simulink model "SWC_FDC_type"  (R2021b)
settings: Solver=FixedStepDiscrete  StartTime=0.0  StopTime=10.0  FixedStep=0.001  RelTol=1e-3
values from neighbouring files (symbols this model uses):
  DID_VCUKey = uint16(0x0202)    [vcu_local_hdr.m]
  DID_XWD = uint16(513)    [vcu_local_hdr.m]
  DIDLen_APSFunConfig = uint16(16)    [vcu_local_hdr.m]
  DIDLen_AutoLock = uint16(1)    [vcu_local_hdr.m]
  DIDLen_DKCKey = uint16(8)    [vcu_local_hdr.m]
  DIDLen_DRLDis = uint16(1)    [vcu_local_hdr.m]
  DIDLen_DynoMode = uint16(1)    [vcu_local_hdr.m]
  DIDLen_FMHTimer = uint16(1)    [vcu_local_hdr.m]
  DIDLen_LFLowPresThre = uint16(1)    [vcu_local_hdr.m]
  DIDLen_LFSensorID = uint16(4)    [vcu_local_hdr.m]
  DIDLen_LRLowPresThre = uint16(1)    [vcu_local_hdr.m]
  DIDLen_LRSensorID = uint16(4)    [vcu_local_hdr.m]
  DIDLen_RFLowPresThre = uint16(1)    [vcu_local_hdr.m]
  DIDLen_RFSensorID = uint16(4)    [vcu_local_hdr.m]
  DIDLen_RRLowPresThre = uint16(1)    [vcu_local_hdr.m]
  DIDLen_RRSensorID = uint16(4)    [vcu_local_hdr.m]
  DIDLen_SensorMode = uint16(1)    [vcu_local_hdr.m]
  DIDLen_TireSize = uint16(16)    [vcu_local_hdr.m]
  DIDLen_TPMSLearnSta = uint16(1)    [vcu_local_hdr.m]
  DIDLen_TurnLampFLThreCurr = uint16(1)    [vcu_local_hdr.m]
  DIDLen_TurnLampFRThreCurr = uint16(1)    [vcu_local_hdr.m]
  DIDLen_TurnLampRLThreCurr = uint16(1)    [vcu_local_hdr.m]
  DIDLen_TurnLampRRThreCurr = uint16(1)    [vcu_local_hdr.m]
  DIDLen_USSConfig = uint16(16)    [vcu_local_hdr.m]
  DIDLen_WhlPres = uint16(4)    [vcu_local_hdr.m]
  DIDLen_WhlSensorBattSta = uint16(1)    [vcu_local_hdr.m]
  DIDLen_WhlTmp = uint16(4)    [vcu_local_hdr.m]
  DIDLen_XWDMode = uint16(1)    [vcu_local_hdr.m]
  DIDNum_APSFunConfig = uint16(0x0903)    [vcu_local_hdr.m]
  DIDNum_AutoLock = uint16(0x0306)    [vcu_local_hdr.m]
  DIDNum_DKCKey = uint16(0x0202)    [vcu_local_hdr.m]
  DIDNum_DRLDis = uint16(0x0307)    [vcu_local_hdr.m]
  DIDNum_DynoMode = uint16(0x0203)    [vcu_local_hdr.m]
  DIDNum_FMHTimer = uint16(0x0305)    [vcu_local_hdr.m]
  DIDNum_LFLowPresThre = uint16(0x0B08)    [vcu_local_hdr.m]
  DIDNum_LFSensorID = uint16(0x0B01)    [vcu_local_hdr.m]
  DIDNum_LRLowPresThre = uint16(0x0B0A)    [vcu_local_hdr.m]
  DIDNum_LRSensorID = uint16(0x0B03)    [vcu_local_hdr.m]
  DIDNum_RFLowPresThre = uint16(0x0B09)    [vcu_local_hdr.m]
  DIDNum_RFSensorID = uint16(0x0B02)    [vcu_local_hdr.m]
  DIDNum_RRLowPresThre = uint16(0x0B0B)    [vcu_local_hdr.m]
  DIDNum_RRSensorID = uint16(0x0B04)    [vcu_local_hdr.m]
  DIDNum_SensorMode = uint16(0x0B0C)    [vcu_local_hdr.m]
  DIDNum_TireSize = uint16(0x0902)    [vcu_local_hdr.m]
  DIDNum_TPMSLearnSta = uint16(0x0B0D)    [vcu_local_hdr.m]
  DIDNum_TurnLampFLThreCurr = uint16(0x0303)    [vcu_local_hdr.m]
  DIDNum_TurnLampFRThreCurr = uint16(0x0301)    [vcu_local_hdr.m]
  DIDNum_TurnLampRLThreCurr = uint16(0x0304)    [vcu_local_hdr.m]
  DIDNum_TurnLampRRThreCurr = uint16(0x0302)    [vcu_local_hdr.m]
  DIDNum_USSConfig = uint16(0x0901)    [vcu_local_hdr.m]
  DIDNum_WhlPres = uint16(0x0B05)    [vcu_local_hdr.m]
  DIDNum_WhlSensorBattSta = uint16(0x0B07)    [vcu_local_hdr.m]
  DIDNum_WhlTmp = uint16(0x0B06)    [vcu_local_hdr.m]
  DIDNum_XWDMode = uint16(0x0201)    [vcu_local_hdr.m]
  DIDVCUKeyLength = uint16(8)    [vcu_local_hdr.m]
  ENUM_DRIVETRAIN_AWD = uint8(  2  )    [vcu_local_hdr.m]
  ENUM_DRIVETRAIN_FWD = uint8(  1  )    [vcu_local_hdr.m]
  ENUM_DRIVETRAIN_RWD = uint8(  0  )    [vcu_local_hdr.m]
  ENUM_TPMSLearnStatus_LEARNED = uint8(  1  )    [vcu_local_hdr.m]
  ENUM_TPMSLearnStatus_LEARNFAIL = uint8(  2  )    [vcu_local_hdr.m]
  ENUM_TPMSLearnStatus_NOTLEARN = uint8(  0  )    [vcu_local_hdr.m]
  ENUM_TPMSSTA_FAT = uint8(  8  )    [vcu_local_hdr.m]
  ENUM_TPMSSTA_LOWBATTERY = uint8(  2  )    [vcu_local_hdr.m]
  FALSE = boolean( 0 )    [vcu_local_hdr.m]
  ONE_INT = uint8(1)    [vcu_local_hdr.m]
  P_boolean = 0.0    [APPTypes.sldd]
  TRUE = boolean( 1 )    [vcu_local_hdr.m]
  ZERO_FLOAT = single(0)    [vcu_local_hdr.m]
  ZERO_INT = uint8(0)    [vcu_local_hdr.m]
undefined symbols (not defined in the file or in its folder): f32_ApsOutVehSpdSig, KHAL_DKCDecryptEnable_flg_ovrdflg, KHAL_DKCDecryptEnable_flg_ovrdval, KHAL_RandomNumberY1_enum, KHAL_RandomNumberY2_enum, KHAL_RandomNumberY_ovrdflg, KHAL_TPMSRESBUTT_flg_ovrdflg, KHAL_TPMSRESBUTT_flg_ovrdval, R_DIDWriteCDD_CSOP_DIDSet_APSFunConfig, R_DIDWriteCDD_CSOP_DIDSet_AutoLock, R_DIDWriteCDD_CSOP_DIDSet_DKCKey, R_DIDWriteCDD_CSOP_DIDSet_DRLDis, R_DIDWriteCDD_CSOP_DIDSet_DynoMode, R_DIDWriteCDD_CSOP_DIDSet_FMHTimer, R_DIDWriteCDD_CSOP_DIDSet_LFLowPresThre, R_DIDWriteCDD_CSOP_DIDSet_LFSensorID, R_DIDWriteCDD_CSOP_DIDSet_LRLowPresThre, R_DIDWriteCDD_CSOP_DIDSet_LRSensorID, R_DIDWriteCDD_CSOP_DIDSet_RFLowPresThre, R_DIDWriteCDD_CSOP_DIDSet_RFSensorID, R_DIDWriteCDD_CSOP_DIDSet_RRLowPresThre, R_DIDWriteCDD_CSOP_DIDSet_RRSensorID, R_DIDWriteCDD_CSOP_DIDSet_SensorMode, R_DIDWriteCDD_CSOP_DIDSet_TireSize, R_DIDWriteCDD_CSOP_DIDSet_TPMSLearnSta, R_DIDWriteCDD_CSOP_DIDSet_TurnLampFLThreCurr, R_DIDWriteCDD_CSOP_DIDSet_TurnLampFRThreCurr, R_DIDWriteCDD_CSOP_DIDSet_TurnLampRLThreCurr, R_DIDWriteCDD_CSOP_DIDSet_TurnLampRRThreCurr, R_DIDWriteCDD_CSOP_DIDSet_USSConfig, R_DIDWriteCDD_CSOP_DIDSet_WhlPres, R_DIDWriteCDD_CSOP_DIDSet_WhlSensorBattSta, R_DIDWriteCDD_CSOP_DIDSet_WhlTmp, R_DIDWriteCDD_CSOP_DIDSet_XWDMode, R_E2E_CAN3_VCU1_CSOP_Write_CAN3_VCU1, R_E2E_CAN3_VCU1_toNIDEC_CSOP_Write_CAN3_VCU1_toNIDEC, R_E2E_CAN4_VCU1_CSOP_Write_CAN4_VCU1, R_FDCCDD_Inner_CSOP_FDC_AppCallSleep, R_HALINCDD_CSOP_PAS_Handler, R_HALINCDD_CSOP_UDS_Main, R_HALOUT_APS_CSOP_ApsOutput, R_HALOUTCDD_CSOP_AppNmStateReq, R_HALOUTCDD_CSOP_SetAcoreRebootCmdACK, R_HALOUTCDD_CSOP_SetSysPwrStat, R_HALOUTCDD_CSOP_SleepRequest, R_IOExpOUT_CDD_CSOP_IOExpSetVal, R_J1939_CAN1_CFGEM1_BAM_CSOP_Write_CAN1_CFGEM1_BAM, R_J1939_CAN1_CFGEM1_DT_CSOP_Write_CAN1_CFGEM1_DT, R_NVMReadCDD_Inner_NVM_ReadOperation, R_NVMWriteCDD_Inner_NVM_WriteOperation, R_UDSCDD_CSOP_DdmRestartOperationCycle, R_WDGCDD_CSOP_Call_Watchdog, R_WDGCDD_CSOP_Call_WDG_AppEnd, R_WDGCDD_CSOP_Call_WDG_AppStart, u16_DIDLen_APSFunConfig, u16_DIDLen_AutoLock, u16_DIDLen_DKCKey, u16_DIDLen_DRLDis, u16_DIDLen_DynoMode, u16_DIDLen_FMHTimer ... (+83)
libraries: simulink x215, FVT_lib x143, hcu_lib x19, hdlsllib x9, app x1, halin x1, halout x1, inp x1, outp x1
(part 3 of 13)

== system SWC_FDC_type/run_SWC_FDC_Tx_10ms_sys ==
  IRV_ms10_CAN1_SG_EMRC1_read : Inport
  IRV_ms10_CAN1_SG_VCU_PDU_Demand_1_read : Inport  Port=2
  IRV_ms10_CAN2_SG_GW2_C10_0_read : Inport  Port=3
  IRV_ms10_CAN3_SG_FD3_VCU0_read : Inport  Port=4
  IRV_ms10_CAN3_SG_FD3_VCU2_read : Inport  Port=5
  IRV_ms10_CAN3_SG_FD3_VCU2_toNIDEC_read : Inport  Port=6
  IRV_ms10_CAN3_SG_FD3_VCU5_read : Inport  Port=7
  IRV_f32_ApsOutVehSpdSig_read : Inport  Port=8
  IRV_u8_ApsOutGearPosnSig_read : Inport  Port=9
  IRV_u8_ApsOutSendChrgPlugSta_read : Inport  Port=10
  IRV_u8_ApsOutSetFrSensorOnCmd_read : Inport  Port=11
  IRV_u8_ApsOutSetFrSensorSwTOCmd_read : Inport  Port=12
  IRV_u8_ApsOutSetVehSpdTOCmd_read : Inport  Port=13
  function : TriggerPort  TriggerType=function-call  VariantControl=(inherit)  SampleTimeType=periodic  SampleTime=-1
  R_HALINCDD_CSOP_TPMS_GetRawData : FunctionCaller  FunctionPrototype=[u8_TPMSDataInSta,u8Array9_TPMSData] = R_HALINCDD_CSOP_TPMS_GetRawData()  OutputArgumentSpecifications=P_boolean, uint8([1;1;1;1;1;1;1;1;1])
  R_HALIN_APS_CSOP_ApsGetDist : FunctionCaller  FunctionPrototype=[u8Array8_PasInDist,u16Array4_ApsInDist] = R_HALIN_APS_CSOP_ApsGetDist()  OutputArgumentSpecifications=uint8([1;1;1;1;1;1;1;1]), uint16([1;1;1;1])
  R_HALIN_APS_CSOP_ApsGetDistLevel : FunctionCaller  FunctionPrototype=u8Array8_ApsInLevel = R_HALIN_APS_CSOP_ApsGetDistLevel()  OutputArgumentSpecifications=uint8([1;1;1;1;1;1;1;1])
  R_HALIN_APS_CSOP_ApsGetOtherStatus : FunctionCaller  FunctionPrototype=[u8_ApsInPASChime,u8_ApsInSensorLayout,u8_ApsInSysFailSta,u8_ApsInSysMode] = R_HALIN_APS_CSOP_ApsGetOtherStatus()  OutputArgumentSpecifications=uint8(1), uint8(1), uint8(1), uint8(1)
  R_HALIN_APS_CSOP_ApsGetUssSta : FunctionCaller  FunctionPrototype=u8Array12_ApsInUssSta = R_HALIN_APS_CSOP_ApsGetUssSta()  OutputArgumentSpecifications=uint8([1;1;1;1;1;1;1;1;1;1;1;1])
  R_HALOUT_APS_CSOP_ApsOutput : FunctionCaller  FunctionPrototype=R_HALOUT_APS_CSOP_ApsOutput(f32_ApsOutVehSpdSig,u8_ApsOutGearPosnSig,u8_ApsOutSetFrSensorOnCmd,u8_ApsOutSetVehSpdTOCmd,u8_ApsOutSetFrSensorSwTOCmd,u8_ApsOutSendChrgPlugSta)  InputArgumentSpecifications=single(1), uint8(1), uint8(1), uint8(1), uint8(1), uint8(1)
  P_CAN1_EMRC1_CAN1_SG_EMRC1_write : Outport
  P_CAN1_VCU_PDU_Demand_1_CAN1_SG_VCU_PDU_Demand_1_write : Outport  Port=2
  P_CAN2_GW2_C10_0_CAN2_SG_GW2_C10_0_write : Outport  Port=3
  P_CAN3_FD3_VCU0_CAN3_SG_FD3_VCU0_write : Outport  Port=4
  P_CAN3_FD3_VCU2_CAN3_SG_FD3_VCU2_write : Outport  Port=5
  P_CAN3_FD3_VCU2_toNIDEC_CAN3_SG_FD3_VCU2_toNIDEC_write : Outport  Port=6
  P_CAN3_FD3_VCU5_CAN3_SG_FD3_VCU5_write : Outport  Port=7
  IRV_u16Array4_ApsInDist_write : Outport  Port=8  OutDataTypeStr=uint16  PortDimensions=4
  IRV_u8Array12_ApsInUssSta_write : Outport  Port=9  OutDataTypeStr=uint8  PortDimensions=12
  IRV_u8Array8_ApsInLevel_write : Outport  Port=10  OutDataTypeStr=uint8  PortDimensions=8
  IRV_u8Array8_PasInDist_write : Outport  Port=11  OutDataTypeStr=uint8  PortDimensions=8
  IRV_u8Array9_TPMSData_write : Outport  Port=12  OutDataTypeStr=uint8  PortDimensions=9
  IRV_u8_ApsInPASChime_write : Outport  Port=13  OutDataTypeStr=uint8  PortDimensions=1
  IRV_u8_ApsInSensorLayout_write : Outport  Port=14  OutDataTypeStr=uint8  PortDimensions=1
  IRV_u8_ApsInSysFailSta_write : Outport  Port=15  OutDataTypeStr=uint8  PortDimensions=1
  IRV_u8_ApsInSysMode_write : Outport  Port=16  OutDataTypeStr=uint8  PortDimensions=1
  IRV_u8_TPMSDataInSta_write : Outport  Port=17  OutDataTypeStr=uint8  PortDimensions=1
  wires:
  R_HALIN_APS_CSOP_ApsGetDist/1 -> IRV_u8Array8_PasInDist_write/1
  R_HALIN_APS_CSOP_ApsGetDist/2 -> IRV_u16Array4_ApsInDist_write/1
  R_HALIN_APS_CSOP_ApsGetDistLevel/1 -> IRV_u8Array8_ApsInLevel_write/1
  R_HALIN_APS_CSOP_ApsGetUssSta/1 -> IRV_u8Array12_ApsInUssSta_write/1
  IRV_f32_ApsOutVehSpdSig_read/1 -> R_HALOUT_APS_CSOP_ApsOutput/1
  IRV_u8_ApsOutGearPosnSig_read/1 -> R_HALOUT_APS_CSOP_ApsOutput/2
  IRV_u8_ApsOutSetFrSensorOnCmd_read/1 -> R_HALOUT_APS_CSOP_ApsOutput/3
  IRV_u8_ApsOutSetVehSpdTOCmd_read/1 -> R_HALOUT_APS_CSOP_ApsOutput/4
  IRV_u8_ApsOutSetFrSensorSwTOCmd_read/1 -> R_HALOUT_APS_CSOP_ApsOutput/5
  IRV_u8_ApsOutSendChrgPlugSta_read/1 -> R_HALOUT_APS_CSOP_ApsOutput/6
  R_HALIN_APS_CSOP_ApsGetOtherStatus/1 -> IRV_u8_ApsInPASChime_write/1
  R_HALIN_APS_CSOP_ApsGetOtherStatus/2 -> IRV_u8_ApsInSensorLayout_write/1
  R_HALIN_APS_CSOP_ApsGetOtherStatus/3 -> IRV_u8_ApsInSysFailSta_write/1
  R_HALIN_APS_CSOP_ApsGetOtherStatus/4 -> IRV_u8_ApsInSysMode_write/1
  R_HALINCDD_CSOP_TPMS_GetRawData/1 -> IRV_u8_TPMSDataInSta_write/1
  R_HALINCDD_CSOP_TPMS_GetRawData/2 -> IRV_u8Array9_TPMSData_write/1
  IRV_ms10_CAN1_SG_EMRC1_read/1 -> P_CAN1_EMRC1_CAN1_SG_EMRC1_write/1
  IRV_ms10_CAN1_SG_VCU_PDU_Demand_1_read/1 -> P_CAN1_VCU_PDU_Demand_1_CAN1_SG_VCU_PDU_Demand_1_write/1
  IRV_ms10_CAN2_SG_GW2_C10_0_read/1 -> P_CAN2_GW2_C10_0_CAN2_SG_GW2_C10_0_write/1
  IRV_ms10_CAN3_SG_FD3_VCU0_read/1 -> P_CAN3_FD3_VCU0_CAN3_SG_FD3_VCU0_write/1
  IRV_ms10_CAN3_SG_FD3_VCU2_toNIDEC_read/1 -> P_CAN3_FD3_VCU2_toNIDEC_CAN3_SG_FD3_VCU2_toNIDEC_write/1
  IRV_ms10_CAN3_SG_FD3_VCU5_read/1 -> P_CAN3_FD3_VCU5_CAN3_SG_FD3_VCU5_write/1
  IRV_ms10_CAN3_SG_FD3_VCU2_read/1 -> P_CAN3_FD3_VCU2_CAN3_SG_FD3_VCU2_write/1

== system SWC_FDC_type/run_SWC_FDC_Tx_20ms_sys ==
  IRV_ms20_CAN2_SG_FD2_C20_0_read : Inport
  function : TriggerPort  TriggerType=function-call  VariantControl=(inherit)  SampleTimeType=periodic  SampleTime=-1
  P_CAN2_FD2_C20_0_CAN2_SG_FD2_C20_0_write : Outport
  wires:
  IRV_ms20_CAN2_SG_FD2_C20_0_read/1 -> P_CAN2_FD2_C20_0_CAN2_SG_FD2_C20_0_write/1

== system SWC_FDC_type/run_SWC_FDC_Tx_250ms_sys ==
  IRV_ms250_CAN1_SG_EEC3_read : Inport
  function : TriggerPort  TriggerType=function-call  VariantControl=(inherit)  SampleTimeType=periodic  SampleTime=-1
  P_CAN1_EEC3_CAN1_SG_EEC3_write : Outport
  wires:
  IRV_ms250_CAN1_SG_EEC3_read/1 -> P_CAN1_EEC3_CAN1_SG_EEC3_write/1

== system SWC_FDC_type/run_SWC_FDC_Tx_5000ms_sys ==
  IRV_ms5000_CAN2_SG_FD2_Version_read : Inport
  function : TriggerPort  TriggerType=function-call  VariantControl=(inherit)  SampleTimeType=periodic  SampleTime=-1
  P_CAN2_FD2_Version_CAN2_SG_FD2_Version_write : Outport
  wires:
  IRV_ms5000_CAN2_SG_FD2_Version_read/1 -> P_CAN2_FD2_Version_CAN2_SG_FD2_Version_write/1

== system SWC_FDC_type/run_SWC_FDC_Tx_50ms_sys ==
  IRV_ms50_CAN1_SG_EEC2_read : Inport
  IRV_ms50_CAN1_SG_ETC2_read : Inport  Port=2
  function : TriggerPort  TriggerType=function-call  VariantControl=(inherit)  SampleTimeType=periodic  SampleTime=-1
  P_CAN1_EEC2_CAN1_SG_EEC2_write : Outport
  P_CAN1_ETC2_CAN1_SG_ETC2_write : Outport  Port=2
  wires:
  IRV_ms50_CAN1_SG_EEC2_read/1 -> P_CAN1_EEC2_CAN1_SG_EEC2_write/1
  IRV_ms50_CAN1_SG_ETC2_read/1 -> P_CAN1_ETC2_CAN1_SG_ETC2_write/1

== system SWC_FDC_type/run_SWC_FDC_Tx_80ms_sys ==
  IRV_ms80_CAN1_SG_ETC1_read : Inport
  function : TriggerPort  TriggerType=function-call  VariantControl=(inherit)  SampleTimeType=periodic  SampleTime=-1
  P_CAN1_ETC1_CAN1_SG_ETC1_write : Outport
  wires:
  IRV_ms80_CAN1_SG_ETC1_read/1 -> P_CAN1_ETC1_CAN1_SG_ETC1_write/1

== system SWC_FDC_type/run_SWC_FDC_UDS_10ms_sys ==
  function : TriggerPort  TriggerType=function-call  VariantControl=(inherit)  SampleTimeType=periodic  SampleTime=-1
  R_HALINCDD_CSOP_UDS_Main : FunctionCaller  FunctionPrototype=R_HALINCDD_CSOP_UDS_Main()

== system SWC_FDC_type/P_WDGCDD/run_SWC_FDC_AppCallWDG_End_sys ==
  function : TriggerPort  TriggerType=function-call  IsSimulinkFunction=on  FunctionName=run_SWC_FDC_AppCallWDG_End  VariantControl=(inherit)

== system SWC_FDC_type/P_WDGCDD/run_SWC_FDC_AppCallWDG_StartUp_sys ==
  function : TriggerPort  TriggerType=function-call  IsSimulinkFunction=on  FunctionName=run_SWC_FDC_AppCallWDG_StartUp  VariantControl=(inherit)

== system SWC_FDC_type/P_WDGCDD/run_SWC_FDC_AppCallWDG_sys ==
  function : TriggerPort  TriggerType=function-call  IsSimulinkFunction=on  FunctionName=run_SWC_FDC_AppCallWDG  VariantControl=(inherit)

== system SWC_FDC_type/run_SWC_FDC_RxTx_5ms_sys/HALOUT_AFTER ==
  E2E_CAN3_VCU1_Trigger : Inport
  E2E_CAN3_VCU1_Trigger_toNIDEC : Inport  Port=2
  E2E_CAN4_VCU1_Trigger : Inport  Port=3
  function : TriggerPort  TriggerType=function-call  VariantControl=(inherit)  PortDimensions=1
  R_E2E_CAN3_VCU1_CSOP_Write_CAN3_VCU1 : Subsystem
  R_E2E_CAN3_VCU1_toNIDEC_CSOP_Write_CAN3_VCU1_toNIDEC : Subsystem
  R_E2E_CAN4_VCU1_CSOP_Write_CAN4_VCU1 : Subsystem
  wires:
  E2E_CAN3_VCU1_Trigger/1 -> R_E2E_CAN3_VCU1_CSOP_Write_CAN3_VCU1/Enable
  E2E_CAN3_VCU1_Trigger_toNIDEC/1 -> R_E2E_CAN3_VCU1_toNIDEC_CSOP_Write_CAN3_VCU1_toNIDEC/Enable
  E2E_CAN4_VCU1_Trigger/1 -> R_E2E_CAN4_VCU1_CSOP_Write_CAN4_VCU1/Enable

== system SWC_FDC_type/run_SWC_FDC_RxTx_5ms_sys/Halin_CDD ==
  PASDistanceData : Inport
  APSDistanceData : Inport  Port=2
  APSLevelData : Inport  Port=3
  APSFaultStaData : Inport  Port=4
  ChimeIn : Inport  Port=5
  SNSRLayoutIn : Inport  Port=6
  StaFSyaIn : Inport  Port=7
  ModOperationIn : Inport  Port=8
  VHAL_AccelPedal1Vol_Raw : Inport  Port=9
  VHAL_AccelPedal2Vol_Raw : Inport  Port=10
  VHAL_BrakeSWGPIO_flg : Inport  Port=11
  VHAL_HoodSW_flg : Inport  Port=12
  VHAL_TailgateSW_flg : Inport  Port=13
  VHAL_DrDoorSW_flg : Inport  Port=14
  VHAL_PsDoorSW_flg : Inport  Port=15
  VHAL_RRDoorSW_flg : Inport  Port=16
  VHAL_RLDoorSW_flg : Inport  Port=17
  VHAL_CentralDoorLockSW_flg : Inport  Port=18
  VHAL_HazardSW_flg : Inport  Port=19
  VHAL_BrakeLampSW_flg : Inport  Port=20
  VHAL_TrunkHanSW_flg : Inport  Port=21
  VHAL_SeatSW_flg : Inport  Port=22
  VHAL_CrashSignalGPIO_flg : Inport  Port=23
  u8_HWID_4byte : Inport  Port=24
  GetSWID_status : Inport  Port=25
  GetSWID_data : Inport  Port=26
  VHAL_AnyNMID_flg : Inport  Port=27
  VHAL_CurrentNmState_enum : Inport  Port=28
  VHAL_PwrReq_OTA_enum : Inport  Port=29
  VHAL_AllowMovThd_OTA_enum : Inport  Port=30
  VHAL_EvccAplusPwrUpReq_flg : Inport  Port=31
  VHAL_AcoreReadyToSlp_flg : Inport  Port=32
  VHAL_DidXWDSta_flg : Inport  Port=33
  VHAL_DidXWDData_enum : Inport  Port=34
  HAL_NvmReadData_raw : Inport  Port=35
  VHAL_DIDVCUKeyReadSta_flg : Inport  Port=36
  VHAL_GetDIDVCUKey_enum : Inport  Port=37
  TPMS_DataIn_flg : Inport  Port=38
  TPMS_RawData : Inport  Port=39
  BHAL_CAN2_outputs : Inport  Port=40
  BHAL_CAN4_outputs : Inport  Port=41
  VHAL_ClearDTCcmd_flg : Inport  Port=42
  VHAL_IMUOffsetVal_raw : Inport  Port=43
  VHAL_IMUSixAxisVal_raw : Inport  Port=44
  VHAL_IMUOffsetValSta_flg : Inport  Port=45
  VHAL_IMUSixAxisValSta_flg : Inport  Port=46
  VHAL_NvmProtectSta_flg : Inport  Port=47
  VHAL_AuxBattVolmV_100mV : Inport  Port=48
  VHAL_Pedal1Ref5V_raw : Inport  Port=49
  VHAL_Pedal2Ref5V_raw : Inport  Port=50
  VHAL_NetworkReqCalled_flg : Inport  Port=51
  VHAL_PmicBootReason_enum : Inport  Port=52
  VHAL_WisrBootReason_raw32 : Inport  Port=53
  BHAL_DIDGetData_raw : Inport  Port=54
  VHAL_AcoreRebootCmd_raw : Inport  Port=55
  VHAL_CAN1BusOff_raw : Inport  Port=56
  VHAL_CAN2BusOff_raw : Inport  Port=57
  VHAL_CAN3BusOff_raw : Inport  Port=58
  VHAL_CAN4BusOff_raw : Inport  Port=59
  VHAL_CAN5BusOff_raw : Inport  Port=60
  u8_GetAPS_Progress_PCT : Inport  Port=61
  u8_GetAPS_RQ_Display : Inport  Port=62
  u8_GetAPS_SW_Ver : Inport  Port=63
  u8_GetAPS_HW_Ver : Inport  Port=64
  u8_GetAPS_ExitCondition : Inport  Port=65
  f32_GetAPS_Angle_Target : Inport  Port=66
  u8_GetAPS_Sta_System : Inport  Port=67
  u8_GetAPS_V_Rq_EPAS_Ctrl : Inport  Port=68
  u8_GetAPS_Rq_EPAS_Ctrl : Inport  Port=69
  u8_GetAPS_Req : Inport  Port=70
  f32_GetAPS_DecReq : Inport  Port=71
  u8_GetAPS_DecReq_A : Inport  Port=72
  f32_GetAPS_SpeedCmd : Inport  Port=73
  u8_GetAPS_ShftPosnReq : Inport  Port=74
  u8_GetAPS_VMC_Req_A : Inport  Port=75
  u8_GetCAAS_Sta : Inport  Port=76
  u8_GetCAAS_VMC_Req_A : Inport  Port=77
  trig_HalinCDD : TriggerPort  TriggerType=function-call  VariantControl=(inherit)
  Halin_APM : Subsystem
  Halin_DKC_A : Subsystem
  Halin_GPIO : Subsystem
  Halin_IMU : Subsystem
  Halin_SYS : Subsystem
  Halin_TPMS : Subsystem
  Subsystem : Subsystem
  TPM_Scheduler : Stateflow chart  TreatAsAtomicUnit=on
  BHAL_APM_outputs : Outport
  BHAL_GPIO_outputs : Outport  Port=2
  BHAL_SYS_outputs : Outport  Port=3
  BHAL_TPMS_outputs : Outport  Port=4
  BHAL_SYSTPMS_outputs : Outport  Port=5
  BHAL_DDM_outputs : Outport  Port=6
  BHAL_IMU_outputs : Outport  Port=7
  Enable_decrypt : Outport  Port=8
  AESKey : Outport  Port=9
  DKCRawData : Outport  Port=10
  wires:
  Halin_DKC_A/1(Enable_Decrypt) -> Enable_decrypt/1
  VHAL_RLDoorSW_flg/1 -> Halin_GPIO/9(VHAL_RLDoorSW_flg)
  Halin_SYS/1(BHAL_SYS_outputs) -> [BHAL_SYS_outputs], BHAL_SYS_outputs/1
  Halin_DKC_A/3(DKCRawData) -> DKCRawData/1
  GetSWID_data/1 -> Halin_SYS/2(GetSWID_data)
  VHAL_GetDIDVCUKey_enum/1 -> Halin_SYS/13(VHAL_GetDIDVCUKey_enum)
  VHAL_TailgateSW_flg/1 -> Halin_GPIO/5(VHAL_TailgateSW_flg)
  Halin_DKC_A/2(AESKey) -> AESKey/1
  VHAL_AccelPedal2Vol_Raw/1 -> Halin_GPIO/2(VHAL_AccelPedal2Vol_Raw)
  TPM_Scheduler/1(trig_TPM_10ms1()) -> Halin_TPMS/Trigger
  VHAL_TrunkHanSW_flg/1 -> Halin_GPIO/13(VHAL_TrunkHanSW_flg)
  VHAL_DidXWDSta_flg/1 -> Halin_SYS/9(VHAL_DidXWDSta_flg)
  VHAL_CurrentNmState_enum/1 -> Halin_SYS/4(VHAL_CurrentNmState_enum)
  VHAL_AccelPedal1Vol_Raw/1 -> Halin_GPIO/1(VHAL_AccelPedal1Vol_Raw)
  u8_HWID_4byte/1 -> Halin_GPIO/16(u8_HWID_4byte)
  BHAL_CAN2_outputs/1 -> Halin_TPMS/3(BHAL_CAN2_outputs)
  VHAL_AcoreReadyToSlp_flg/1 -> Halin_SYS/8(VHAL_AcoreReadyToSlp_flg)
  HAL_NvmReadData_raw/1 -> Halin_SYS/11(HAL_NvmReadData_raw)
  VHAL_AllowMovThd_OTA_enum/1 -> Halin_SYS/6(VHAL_AllowMovThd_OTA_enum)
  VHAL_BrakeLampSW_flg/1 -> Halin_GPIO/12(VHAL_BrakeLampSW_flg)
  VHAL_RRDoorSW_flg/1 -> Halin_GPIO/8(VHAL_RRDoorSW_flg)
  VHAL_BrakeSWGPIO_flg/1 -> Halin_GPIO/3(VHAL_BrakeSWGPIO_flg)
  GetSWID_status/1 -> Halin_SYS/1(GetSWID_status)
  VHAL_DrDoorSW_flg/1 -> Halin_GPIO/6(VHAL_DrDoorSW_flg)
  VHAL_PwrReq_OTA_enum/1 -> Halin_SYS/5(VHAL_PwrReq_OTA_enum)
  VHAL_HoodSW_flg/1 -> Halin_GPIO/4(VHAL_HoodSW_flg)
  Halin_GPIO/1(BHAL_GPIO_outputs) -> BHAL_GPIO_outputs/1
  BHAL_CAN4_outputs/1 -> Halin_DKC_A/1(BHAL_CAN4_outputs)
  VHAL_CentralDoorLockSW_flg/1 -> Halin_GPIO/10(VHAL_CentralDoorLockSW_flg)
  TPMS_RawData/1 -> Halin_TPMS/2(TPMS_RawData)
  VHAL_CrashSignalGPIO_flg/1 -> Halin_GPIO/15(VHAL_CrashSignalGPIO_flg)
  Halin_TPMS/1(BHAL_TPMS_outputs) -> BHAL_TPMS_outputs/1
  VHAL_DidXWDData_enum/1 -> Halin_SYS/10(VHAL_DidXWDData_enum)
  VHAL_EvccAplusPwrUpReq_flg/1 -> Halin_SYS/7(VHAL_EvccAplusPwrUpReq_flg)
  VHAL_SeatSW_flg/1 -> Halin_GPIO/14(VHAL_SeatSW_flg)
  VHAL_DIDVCUKeyReadSta_flg/1 -> Halin_SYS/12(VHAL_DIDVCUKeyReadSta_flg)
  VHAL_PsDoorSW_flg/1 -> Halin_GPIO/7(VHAL_PsDoorSW_flg)
  [BHAL_SYS_outputs] -> Halin_DKC_A/2(BHAL_SYS_outputs)
  TPMS_DataIn_flg/1 -> Halin_TPMS/1(TPMS_DataIn_flg)
  VHAL_AnyNMID_flg/1 -> Halin_SYS/3(VHAL_AnyNMID_flg)
  VHAL_HazardSW_flg/1 -> Halin_GPIO/11(VHAL_HazardSW_flg)
  Halin_SYS/2(BHAL_SYSTPMS_outputs) -> [BHAL_SYSTPMS_outputs], BHAL_SYSTPMS_outputs/1
  [BHAL_SYSTPMS_outputs] -> Halin_TPMS/4(BHAL_SYSTPMS_outputs)
  VHAL_ClearDTCcmd_flg/1 -> Subsystem/1(VHAL_ClearDTCcmd_flg)
  Subsystem/1(BHAL_DDM_outputs) -> BHAL_DDM_outputs/1
  Halin_IMU/1(BHAL_IMU_outputs) -> BHAL_IMU_outputs/1
  VHAL_IMUOffsetVal_raw/1 -> Halin_IMU/1(VHAL_IMUOffsetVal_raw)
  VHAL_IMUOffsetValSta_flg/1 -> Halin_IMU/3(VHAL_IMUOffsetValSta_flg)
  VHAL_IMUSixAxisVal_raw/1 -> Halin_IMU/2(VHAL_IMUSixAxisVal_raw)
  VHAL_IMUSixAxisValSta_flg/1 -> Halin_IMU/4(VHAL_IMUSixAxisValSta_flg)
  VHAL_NvmProtectSta_flg/1 -> Halin_SYS/14(VHAL_NvmProtectSta_flg)
  VHAL_AuxBattVolmV_100mV/1 -> Halin_SYS/15(VHAL_AuxBattVolmV_100mV)
  VHAL_Pedal1Ref5V_raw/1 -> Halin_SYS/16(VHAL_Pedal1Ref5V_raw)
  VHAL_Pedal2Ref5V_raw/1 -> Halin_SYS/17(VHAL_Pedal2Ref5V_raw)
  VHAL_NetworkReqCalled_flg/1 -> Halin_SYS/18(VHAL_NetworkReqCalled_flg)
  VHAL_PmicBootReason_enum/1 -> Halin_SYS/19(VHAL_PmicBootReason_enum)
  VHAL_WisrBootReason_raw32/1 -> Halin_SYS/20(VHAL_WisrBootReason_raw32)
  BHAL_DIDGetData_raw/1 -> Halin_SYS/21(BHAL_DIDGetData_raw)
  VHAL_AcoreRebootCmd_raw/1 -> Halin_SYS/22(VHAL_AcoreRebootCmd_raw)
  VHAL_CAN1BusOff_raw/1 -> Halin_SYS/23(VHAL_CAN1BusOff_raw)
  VHAL_CAN2BusOff_raw/1 -> Halin_SYS/24(VHAL_CAN2BusOff_raw)
  VHAL_CAN3BusOff_raw/1 -> Halin_SYS/25(VHAL_CAN3BusOff_raw)
  VHAL_CAN4BusOff_raw/1 -> Halin_SYS/26(VHAL_CAN4BusOff_raw)
  VHAL_CAN5BusOff_raw/1 -> Halin_SYS/27(VHAL_CAN5BusOff_raw)
  Halin_APM/1(BHAL_APM_outputs) -> BHAL_APM_outputs/1
  u8_GetAPS_ShftPosnReq/1 -> Halin_APM/22(u8_GetAPS_ShftPosnReq)
  f32_GetAPS_SpeedCmd/1 -> Halin_APM/21(f32_GetAPS_SpeedCmd)
  f32_GetAPS_Angle_Target/1 -> Halin_APM/14(f32_GetAPS_Angle_Target)
  u8_GetAPS_Sta_System/1 -> Halin_APM/15(u8_GetAPS_Sta_System)
  u8_GetAPS_HW_Ver/1 -> Halin_APM/12(u8_GetAPS_HW_Ver)
  u8_GetAPS_DecReq_A/1 -> Halin_APM/20(u8_GetAPS_DecReq_A)
  u8_GetAPS_Req/1 -> Halin_APM/18(u8_GetAPS_Req)
  u8_GetCAAS_Sta/1 -> Halin_APM/24(u8_GetCAAS_Sta)
  u8_GetAPS_V_Rq_EPAS_Ctrl/1 -> Halin_APM/16(u8_GetAPS_V_Rq_EPAS_Ctrl)
  u8_GetCAAS_VMC_Req_A/1 -> Halin_APM/25(u8_GetCAAS_VMC_Req_A)
  u8_GetAPS_Rq_EPAS_Ctrl/1 -> Halin_APM/17(u8_GetAPS_Rq_EPAS_Ctrl)
  u8_GetAPS_Progress_PCT/1 -> Halin_APM/9(u8_GetAPS_Progress_PCT)
  PASDistanceData/1 -> Halin_APM/1(PASDistanceData)
  u8_GetAPS_ExitCondition/1 -> Halin_APM/13(u8_GetAPS_ExitCondition)
  ChimeIn/1 -> Halin_APM/5(ChimeIn)
  u8_GetAPS_SW_Ver/1 -> Halin_APM/11(u8_GetAPS_SW_Ver)
  APSFaultStaData/1 -> Halin_APM/4(APSFaultStaData)
  u8_GetAPS_RQ_Display/1 -> Halin_APM/10(u8_GetAPS_RQ_Display)
  ModOperationIn/1 -> Halin_APM/8(ModOperationIn)
  APSLevelData/1 -> Halin_APM/3(APSLevelData)
  APSDistanceData/1 -> Halin_APM/2(APSDistanceData)
  StaFSyaIn/1 -> Halin_APM/7(StaFSyaIn)
  f32_GetAPS_DecReq/1 -> Halin_APM/19(f32_GetAPS_DecReq)
  u8_GetAPS_VMC_Req_A/1 -> Halin_APM/23(u8_GetAPS_VMC_Req_A)
  SNSRLayoutIn/1 -> Halin_APM/6(SNSRLayoutIn)

== system SWC_FDC_type/run_SWC_FDC_RxTx_5ms_sys/OUTP_AFTER ==
  BOUTP_outputs : Inport
  BHAL_SYSTPMS_outputs : Inport  Port=2
  BHAL_SYS_outputs : Inport  Port=3
  trig_OUTP_After : TriggerPort  TriggerType=function-call  VariantControl=(inherit)
  APM : Subsystem
  DID_list : Subsystem
  DTC_list : Subsystem  Commented=on
  Subsystem5 : Subsystem
  ApsOut_GearPosnSig : Outport
  ApsOut_SendChrgPlugStaSig : Outport  Port=2
  ApsOut_SetFrSensorOnCmd : Outport  Port=3
  ApsOut_SetFrSensorSwTOCmd : Outport  Port=4
  ApsOut_SetVehSpdTOCmd : Outport  Port=5
  ApsOut_VehSpdSig : Outport  Port=6
  HAL_NvmWriteData_raw : Outport  Port=7
  DTC_Trigger : Outport  Port=8
  Header_Array : Outport  Port=9
  DTC_Array : Outport  Port=10
  BOUTP_DIDSetData_outputs : Outport  Port=11
  wires:
  APM/1(ApsOut_GearPosnSig) -> ApsOut_GearPosnSig/1
  Subsystem5/1(HAL_NvmWriteData_raw) -> HAL_NvmWriteData_raw/1
  APM/2(ApsOut_SendChrgPlugStaSig) -> ApsOut_SendChrgPlugStaSig/1
  APM/5(ApsOut_SetVehSpdTOCmd) -> ApsOut_SetVehSpdTOCmd/1
  APM/3(ApsOut_SetFrSensorOnCmd) -> ApsOut_SetFrSensorOnCmd/1
  BOUTP_outputs/1 -> [BOUTP_outputs]
  APM/6(ApsOut_VehSpdSig) -> ApsOut_VehSpdSig/1
  APM/4(ApsOut_SetFrSensorSwTOCmd) -> ApsOut_SetFrSensorSwTOCmd/1
  [BOUTP_outputs] -> APM/1(BOUTP_outputs)
  [BOUTP_outputs] -> Subsystem5/1(BOUTP_outputs)
  BHAL_SYSTPMS_outputs/1 -> [BHAL_SYSTPMS_outputs]
  [BHAL_SYSTPMS_outputs] -> Subsystem5/2(BHAL_SYSTPMS_outputs)
  [BOUTP_outputs] -> DTC_list/1(BOUTP_outputs)
  DTC_list/1(Trigger) -> DTC_Trigger/1
  DTC_list/2(Header_Array) -> Header_Array/1
  DTC_list/3(DTC_Array) -> DTC_Array/1
  BHAL_SYS_outputs/1 -> [BHAL_SYS_outputs]
  [BHAL_SYS_outputs] -> Subsystem5/3(BHAL_SYS_outputs)
  [BOUTP_outputs] -> DID_list/1(BOUTP_outputs)
  DID_list/1(BOUTP_DIDSetData_outputs) -> BOUTP_DIDSetData_outputs/1

== system SWC_FDC_type/run_SWC_FDC_RxTx_5ms_sys/R_FDCCDD_Inner_CSOP_FDC_AppCallSleep ==
  Enable : EnablePort
  R_FDCCDD_Inner_CSOP_FDC_AppCallSleep : FunctionCaller  FunctionPrototype=R_FDCCDD_Inner_CSOP_FDC_AppCallSleep()

== system SWC_FDC_type/run_SWC_FDC_RxTx_5ms_sys/R_HALIN_IMU_CSOP_IMUGetOffsetVal ==
  trig_ReadIMUOffset_00 : TriggerPort  TriggerType=function-call  VariantControl=(inherit)  PortDimensions=1
  R_HALIN_IMU_CSOP_IMUGetOffsetVal : FunctionCaller  FunctionPrototype=[s16_IMUOffsetVal,u8_IMUOffsetValSta] = R_HALIN_IMU_CSOP_IMUGetOffsetVal()  OutputArgumentSpecifications=int16([1;1;1;1;1;1]), uint8(1)
  Out1 : Outport
  Out2 : Outport  Port=2
  wires:
  R_HALIN_IMU_CSOP_IMUGetOffsetVal/1 -> Out1/1
  R_HALIN_IMU_CSOP_IMUGetOffsetVal/2 -> Out2/1

== system SWC_FDC_type/run_SWC_FDC_RxTx_5ms_sys/R_HALOUTCDD_CSOP_AppNmStateReq ==
  WakeReq : Inport
  SleepReq : Inport  Port=2
  Enable : EnablePort
  R_HALOUTCDD_CSOP_AppNmStateReq : FunctionCaller  FunctionPrototype=R_HALOUTCDD_CSOP_AppNmStateReq(u8_WakeUpReq,u8_SleepReq)  InputArgumentSpecifications=uint8(1), uint8(1)
  wires:
  SleepReq/1 -> R_HALOUTCDD_CSOP_AppNmStateReq/2
  WakeReq/1 -> R_HALOUTCDD_CSOP_AppNmStateReq/1

== system SWC_FDC_type/run_SWC_FDC_RxTx_5ms_sys/R_HALOUTCDD_CSOP_SetAcoreRebootCmdACK ==
  Enable : EnablePort
  R_HALOUTCDD_CSOP_SetAcoreRebootCmdACK : FunctionCaller  FunctionPrototype=R_HALOUTCDD_CSOP_SetAcoreRebootCmdACK()

== system SWC_FDC_type/run_SWC_FDC_RxTx_5ms_sys/R_HALOUTCDD_CSOP_SleepRequest ==
  SleepState : Inport
  WakeUpTime : Inport  Port=2
  Enable : EnablePort
  R_HALOUTCDD_CSOP_SleepRequest : FunctionCaller  FunctionPrototype=R_HALOUTCDD_CSOP_SleepRequest(u32_SleepyState,u32_Wakeup_Timer_s)  InputArgumentSpecifications=uint32(1), uint32(1)
  wires:
  SleepState/1 -> R_HALOUTCDD_CSOP_SleepRequest/1
  WakeUpTime/1 -> R_HALOUTCDD_CSOP_SleepRequest/2

== system SWC_FDC_type/run_SWC_FDC_RxTx_5ms_sys/R_NVMReadCDD_Inner_NVM_ReadOperation ==
  trig_ReadNVM : TriggerPort  TriggerType=function-call  VariantControl=(inherit)  PortDimensions=1
  R_NVMReadCDD_Inner_NVM_ReadOperation : FunctionCaller  FunctionPrototype=R_NVMReadCDD_Inner_NVM_ReadOperation()

== system SWC_FDC_type/run_SWC_FDC_RxTx_5ms_sys/R_NVMWriteCDD_Inner_NVM_WriteOperation ==
  Enable : EnablePort
  R_NVMWriteCDD_Inner_NVM_WriteOperation : FunctionCaller  FunctionPrototype=R_NVMWriteCDD_Inner_NVM_WriteOperation()

== system SWC_FDC_type/run_SWC_FDC_RxTx_5ms_sys/R_UDSCDD_CSOP_DdmRestartOperationCycle ==
  Enable : EnablePort
  R_UDSCDD_CSOP_DdmRestartOperationCycle : FunctionCaller  FunctionPrototype=R_UDSCDD_CSOP_DdmRestartOperationCycle()

== system SWC_FDC_type/run_SWC_FDC_RxTx_5ms_sys/R_UDSCDD_CSOP_SetDTCStatus ==
  Header_Array : Inport
  DTC_Array : Inport  Port=2
  Enable : EnablePort
  R_UDSCDD_CSOP_SetDTCStatus : FunctionCaller  FunctionPrototype=u8_ReturnStatus = R_UDSCDD_CSOP_SetDTCStatus(u32Array10_Header,u32Array320_DTC)  InputArgumentSpecifications=uint32([1;1;1;1;1;1;1;1;1;1]), uint32([1;1;1;1;1;1;1;1;1;1;1;1;1;1;1;1;1;1;1;1;1;1;1;1;1;1;1;1;1;1;1;1;1;1;1;1;1;1;1;1;1;1;1;1;1;1;1;1;1;1;1;1;1;1;1;1;1;1;1;1;1;1;1;1;1;1;1;1;1;1;1;1;1;1;1;1;1;1;1;1;1;1;1;1;1;1;1;1;1;1;1;1;1;1;1;1;1;1;1;1;1;1;1;1;1;1;1;1;1;1;1;1;1;1;1;1;1;1;1;1;1;1;1;1;1;1;1;1;1;1;1;1;1;1;1;1;1;1;1;1;1;1;1;1;1;1;1;1;1;1;1;1;1;1;1;1;1;1;1;1;1;1;1;1;1;1;1;1;1;1;1;1;1;1;1;1;1;1;1;1;1;1;1;1;1;1;1;1;1;1;1;1;1;1;1;1;1;1;1;1;1;1;1;1;1;1;1;1;1;1;1;1;1;1;1;1;1;1;1;1;1;1;1;1;1;1;1;1;1;1;1;1;1;1;1;1;1;1;1;1;1;1;1;1;1;1;1;1;1;1;1;1;1;1;1;1;1;1;1;1;1;1;1;1;1;1;1;1;1;1;1;1;1;1;1;1;1;1;1;1;1;1;1;1;1;1;1;1;1;1;1;1;1;1;1;1;1;1;1;1;1;1;1;1;1;1;1;1;1;1;1;1;1;1;1;1;1;1;1;1])  OutputArgumentSpecifications=uint8(1)
  Out1 : Outport
  wires:
  DTC_Array/1 -> R_UDSCDD_CSOP_SetDTCStatus/2
  Header_Array/1 -> R_UDSCDD_CSOP_SetDTCStatus/1
  R_UDSCDD_CSOP_SetDTCStatus/1 -> Out1/1

== system SWC_FDC_type/run_SWC_FDC_RxTx_5ms_sys/R_WDGCDD_CSOP_Call_WDG_AppEnd ==
  Enable : EnablePort
  R_WDGCDD_CSOP_Call_WDG_AppEnd : FunctionCaller  FunctionPrototype=R_WDGCDD_CSOP_Call_WDG_AppEnd()

== system SWC_FDC_type/run_SWC_FDC_RxTx_5ms_sys/R_WDGCDD_CSOP_Call_WDG_AppStart ==
  Enable : EnablePort
  R_WDGCDD_CSOP_Call_WDG_AppStart : FunctionCaller  FunctionPrototype=R_WDGCDD_CSOP_Call_WDG_AppStart()

== system SWC_FDC_type/run_SWC_FDC_RxTx_5ms_sys/R_WDGCDD_CSOP_Call_Watchdog ==
  trig_WDG : TriggerPort  TriggerType=function-call  VariantControl=(inherit)  PortDimensions=1
  R_WDGCDD_CSOP_Call_Watchdog : FunctionCaller  FunctionPrototype=R_WDGCDD_CSOP_Call_Watchdog()

== system SWC_FDC_type/run_SWC_FDC_RxTx_5ms_sys/Subsystem ==
  In1 : Inport
  In2 : Inport  Port=2
  function : TriggerPort  TriggerType=function-call  VariantControl=(inherit)
  R_HALINCDD_CSOP_DKCDecrypt : FunctionCaller  FunctionPrototype=u8Array16_ResultData = R_HALINCDD_CSOP_DKCDecrypt(u8Array16_AESkey,u8Array16_RawData)  InputArgumentSpecifications=uint8([1;1;1;1;1;1;1;1;1;1;1;1;1;1;1;1]), uint8([1;1;1;1;1;1;1;1;1;1;1;1;1;1;1;1])  OutputArgumentSpecifications=uint8([1;1;1;1;1;1;1;1;1;1;1;1;1;1;1;1])
  Out1 : Outport
  wires:
  In1/1 -> R_HALINCDD_CSOP_DKCDecrypt/1
  R_HALINCDD_CSOP_DKCDecrypt/1 -> Out1/1
  In2/1 -> R_HALINCDD_CSOP_DKCDecrypt/2

== system SWC_FDC_type/run_SWC_FDC_RxTx_5ms_sys/Subsystem1 ==
  In1 : Inport
  Enable : EnablePort
  R_IOExpOUT_CDD_CSOP_IOExpSetVal : FunctionCaller  FunctionPrototype=R_IOExpOUT_CDD_CSOP_IOExpSetVal(u8_IVIRstCmd)  InputArgumentSpecifications=uint8(1)
  wires:
  In1/1 -> R_IOExpOUT_CDD_CSOP_IOExpSetVal/1

== system SWC_FDC_type/run_SWC_FDC_RxTx_5ms_sys/Subsystem2 ==
  Enable_Decrypt : Inport
  u8Array16_ResultData : Inport  Port=2
  BHAL_CAN4_outputs : Inport  Port=3
  function : TriggerPort  TriggerType=function-call  VariantControl=(inherit)
  DKC2 : Subsystem  AncestorBlock=halin_NA_Ref/HAL_IN/DKC1
  Data Type Conversion97 : DataTypeConversion  OutDataTypeStr=uint8
  BHAL_DKC_outputs : Outport
  wires:
  [u8Array16_ResultData] -> Data Type Conversion97/1
  DKC2/1(BHAL_DKC_outputs) -> BHAL_DKC_outputs/1
  Data Type Conversion97/1 -> DKC2/2(DKC_ResultData_16byte)
  BHAL_CAN4_outputs/1 -> DKC2/3(BHAL_CAN4_outputs)
  Enable_Decrypt/1 -> DKC2/1(Enable_Decrypt)
  u8Array16_ResultData/1 -> [u8Array16_ResultData]
